simulink model "Dynamics"  (R2017a)
settings: Solver=VariableStepAuto  StartTime=0.0  StopTime=10.0  RelTol=1e-3
libraries: simulink x2
settings Model: Creator=ASUS  LastModifiedBy=ASUS
settings DataIOCC: ReturnWorkspaceOutputs=on
settings DebuggingCC: SFMachineParentedDataDiag=error
settings SFSimCC: SimUseLocalCustomCode=on
settings RTWCC: RTWUseLocalCustomCode=on

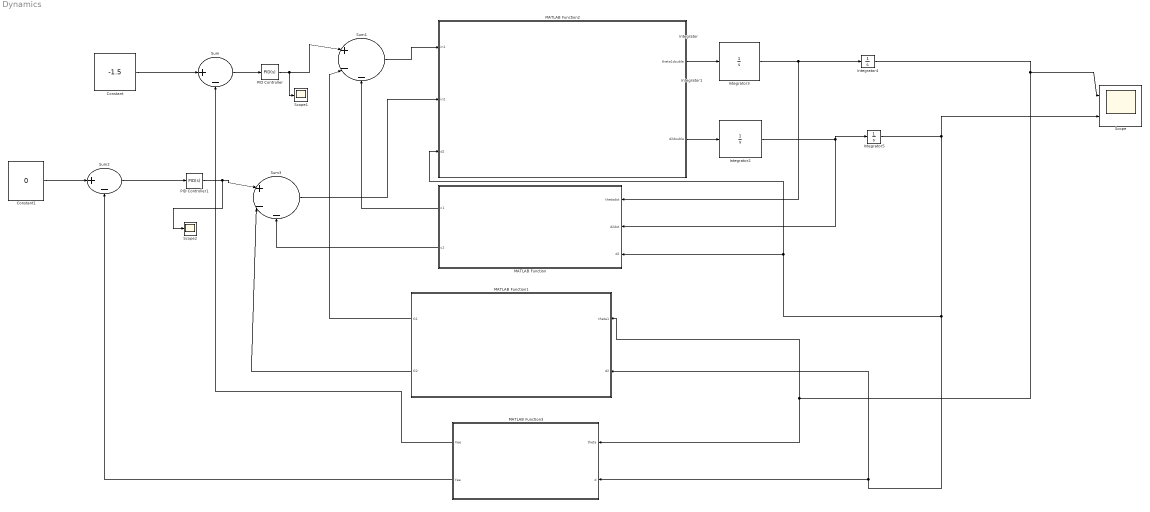
== system Dynamics ==
  Constant : Constant  Value=-1.5
  Constant1 : Constant  Value=0
  Integrator{,1..5} (6 alike) : Integrator
  MATLAB Function : MATLAB Function  TreatAsAtomicUnit=on
  MATLAB Function1 : MATLAB Function  TreatAsAtomicUnit=on
  MATLAB Function2 : MATLAB Function  TreatAsAtomicUnit=on
  MATLAB Function3 : MATLAB Function  TreatAsAtomicUnit=on
  PID Controller : simulink/Continuous/PID Controller  Controller=PID  Form=Parallel  TimeDomain=Continuous-time  SampleTime=-1  IntegratorMethod=Forward Euler  ControllerParametersSource=internal  P=1  I=1  D=0  UseFilter=on  N=100  InitialConditionSource=internal  InitialConditionForIntegrator=0  InitialConditionForFilter=0  DifferentiatorICPrevScaledInput=0  ExternalReset=none  TrackingMode=off  Kt=1  LimitOutput=off  UpperSaturationLimit=inf  LowerSaturationLimit=-inf  LinearizeAsGain=on  AntiWindupMode=none  Kb=1  POutMin=[]  POutMax=[]  IOutMin=[]  IOutMax=[]  DOutMin=[]  DOutMax=[]  NOutMin=[]  NOutMax=[]  SumOutMin=[]  SumOutMax=[]  SaturationOutMin=[]  SaturationOutMax=[]  PParamMin=[]  PParamMax=[]  IParamMin=[]  IParamMax=[]  DParamMin=[]  DParamMax=[]  NParamMin=[]  NParamMax=[]  KbParamMin=[]  KbParamMax=[]  KtParamMin=[]  KtParamMax=[]  KbOutMin=[]  KbOutMax=[]  KtOutMin=[]  KtOutMax=[]  IntegratorOutMin=[]  IntegratorOutMax=[]  FilterOutMin=[]  FilterOutMax=[]  SumI1OutMin=[]  SumI1OutMax=[]  SumI2OutMin=[]  SumI2OutMax=[]  SumI3OutMin=[]  SumI3OutMax=[]  SumDOutMin=[]  SumDOutMax=[]  DifferentiatorOutMin=[]  DifferentiatorOutMax=[]  IntegratorContinuousStateAttributes=''  IntegratorStateMustResolveToSignalObject=off  IntegratorRTWStateStorageClass=Auto  FilterContinuousStateAttributes=''  FilterStateMustResolveToSignalObject=off  FilterRTWStateStorageClass=Auto  InitialConditionSetting=State (most efficient)
  PID Controller1 : simulink/Continuous/PID Controller  Controller=PID  Form=Parallel  TimeDomain=Continuous-time  SampleTime=-1  IntegratorMethod=Forward Euler  ControllerParametersSource=internal  P=1  I=1  D=0  UseFilter=on  N=100  InitialConditionSource=internal  InitialConditionForIntegrator=0  InitialConditionForFilter=0  DifferentiatorICPrevScaledInput=0  ExternalReset=none  TrackingMode=off  Kt=1  LimitOutput=off  UpperSaturationLimit=inf  LowerSaturationLimit=-inf  LinearizeAsGain=on  AntiWindupMode=none  Kb=1  POutMin=[]  POutMax=[]  IOutMin=[]  IOutMax=[]  DOutMin=[]  DOutMax=[]  NOutMin=[]  NOutMax=[]  SumOutMin=[]  SumOutMax=[]  SaturationOutMin=[]  SaturationOutMax=[]  PParamMin=[]  PParamMax=[]  IParamMin=[]  IParamMax=[]  DParamMin=[]  DParamMax=[]  NParamMin=[]  NParamMax=[]  KbParamMin=[]  KbParamMax=[]  KtParamMin=[]  KtParamMax=[]  KbOutMin=[]  KbOutMax=[]  KtOutMin=[]  KtOutMax=[]  IntegratorOutMin=[]  IntegratorOutMax=[]  FilterOutMin=[]  FilterOutMax=[]  SumI1OutMin=[]  SumI1OutMax=[]  SumI2OutMin=[]  SumI2OutMax=[]  SumI3OutMin=[]  SumI3OutMax=[]  SumDOutMin=[]  SumDOutMax=[]  DifferentiatorOutMin=[]  DifferentiatorOutMax=[]  IntegratorContinuousStateAttributes=''  IntegratorStateMustResolveToSignalObject=off  IntegratorRTWStateStorageClass=Auto  FilterContinuousStateAttributes=''  FilterStateMustResolveToSignalObject=off  FilterRTWStateStorageClass=Auto  InitialConditionSetting=State (most efficient)
  Scope : Scope  NumInputPorts=2
  Scope1 : Scope
  Scope2 : Scope
  Sum : Sum  Inputs=|+-
  Sum1 : Sum  Inputs=|+--
  Sum2 : Sum  Inputs=|+-
  Sum3 : Sum  Inputs=|+--
  wires:
  Constant/1 -> Sum/1
  Constant1/1 -> Sum2/1
  Sum/1 -> PID Controller/1
  Sum2/1 -> PID Controller1/1
  PID Controller1/1 -> Scope2/1, Sum3/1
  PID Controller/1 -> Scope1/1, Sum1/1
  Sum3/1 -> MATLAB Function2/2(in2)
  Sum1/1 -> MATLAB Function2/1(in1)
  MATLAB Function2/1(theta1double) -> Integrator3/1
  Integrator3/1 -> Integrator4/1, MATLAB Function/1(thetadot)
  MATLAB Function2/2(d2double) -> Integrator2/1
  Integrator2/1 -> Integrator5/1, MATLAB Function/2(d2dot)
  Integrator5/1 -> MATLAB Function2/3(d2), MATLAB Function/3(d2), MATLAB Function3/2(d), MATLAB Function1/2(d2), Scope/2
  MATLAB Function/1(c1) -> Sum1/3
  MATLAB Function/2(c2) -> Sum3/3
  Integrator4/1 -> MATLAB Function3/1(theta), MATLAB Function1/1(theta1), Scope/1
  MATLAB Function1/1(G1) -> Sum1/2
  MATLAB Function1/2(G2) -> Sum3/2
  MATLAB Function3/1(Xee) -> Sum/2
  MATLAB Function3/2(Yee) -> Sum2/2

== matlab function Dynamics/MATLAB Function1 ==
  data: theta1 input; G1 output; d2 input; G2 output
function [G1,G2] = fcn_Gravational_Forces(theta1,d2)
m1 =  0.3;
m2 = 0.7;
L1 = 1;
g = 9.8;

G = [((-(m1 * L1 * g)/2)+(m2 * g )*( L1+(d2/2)))*cosd(theta1);((m2*g)/2)*sind(theta1)];

G1 = G (1);
G2 = G (2);

end

== matlab function Dynamics/MATLAB Function ==
  data: thetadot input; c1 output; d2dot input; d2 input; c2 output
function [c1,c2] = fcn_Cetrifugal_Forces(thetadot,d2dot,d2)
m2= 0.7;
L1=1;
CO = ([0 0;-(m2/2)*(L1+(d2/2)) 0]*[thetadot^2;d2dot^2]);
CET = ([(2*m2)*(L1+(d2/2)); 0]*[thetadot*d2dot]);
CE = CO + CET ;
c1 = CE (1);
c2 = CE (2);

end

== matlab function Dynamics/MATLAB Function2 ==
  data: in1 input; theta1double output; in2 input; d2double output; d2 input
function [theta1double,d2double] = fcn_Inertia(in1,in2,d2)

a2 = 0.3;
b1 = 0.04;
b2 = 0.04;
m1 = 0.3;
m2= 0.7;
L1=1;
Iz1=(1/2)*0.3*((a2^2)+(b1^2));
Iz2=(1/2)*0.7*((a2^2)+(b2^2));
MI=[((m1*L1^2)/4)+Iz1+m2*((L1+(d2/2)^2))+Iz2 0;0 (m2/4)];
Dots2 = inv(MI)*[in1;in2];
theta1double = Dots2(1);
d2double = Dots2(2);

end

== matlab function Dynamics/MATLAB Function3 ==
  data: Xee output; theta input; d input; Yee output
function [Xee,Yee] = RP_position_forward_kinematics(theta,d)
L1=0.5;

  Xee = (L1+d)*cosd(theta);
  Yee = (L1+d)*sind(theta);
  
end
